simulink model "EV_Modeling"  (R2024b)
(part 7 of 9)

  " Normalization"/3(Current_n) -> Mux2/3
  " Normalization"/1(Temperature_n) -> Mux2/1
  Mux2/1 -> LSTM/1(sequenceinput)
  Divide12/1 -> Add4/1  "Motor_Current"
  Gain5/1 -> Battery_SOC[%]/1, SOC switch/1  "LSTM_LV"
  SOC-Vol/1 -> Voltage_cell/1, " Normalization"/2(Voltage), Vol-R/1, Divide11/1, Vol_pack/1  "Vsoc"
  Zero-Order Hold/1 -> Extended Kalman Filter/1
  Add4/1 -> Gain17/1
  SOC-Temp/1 -> Temperature_cell/1, " Normalization"/1(Temperature)
  SOC switch/1 -> SOC_t-1/1
  Coulomb Counting/1(SOC_CC) -> SOC switch/3, Zero-Order Hold/1
  Zero-Order Hold1/1 -> Extended Kalman Filter/2
  Divide11/1 -> Add4/2  "electric_consumption_Current"
  Extended Kalman Filter/1 -> Gain5/1
  Sum/1 -> [IVD]
  Divide28/1 -> Divide29/1
  From Workspace20/1 -> Divide34/2
  Add1/1 -> Divide33/1
  Constant13/1 -> Divide26/1
  [T_motor] -> Divide38/1
  Divide29/1 -> [T_motor]
  Signal Specification9/1 -> [Motor_radpsec]
  [IVD] -> Saturation1/1
  Gain20/1 -> [Motor_RPM]
  Delay One Step1/1 -> Divide26/2
  Add13/1 -> Divide25/1
  Divide39/1 -> [Electric_Power]
  Add14/1 -> [F_accel]
  [Speed_ms] -> Divide22/2
  [F_resistance] -> Add11/2
  Divide1/1 -> Add1/2  "Motor_Torque[N.m]"
  Divide26/1 -> Add15/4  "F_accel"
  From Workspace14/1 -> Divide29/2
  Divide23/1 -> Add15/3  "F_aero"
  Brake[%]1/1 -> Divide25/2, Divide2/1
  Unit Conversion4/1 -> Signal Specification9/1
  From Workspace21/1 -> Divide35/3
  Divide35/1 -> Divide36/2
  [Motor_RPM] -> 2-D Lookup Table1/1
  Gain23/1 -> Divide39/2
  Compare To Constant3/1 -> Switch1/2
  Divide37/1 -> Gain20/1
  Divide34/1 -> Add14/2
  BPP[%]*MAX_Brake_Force[N]1/1 -> Add14/1  "Brake_Force"
  Constant12/1 -> Divide23/3
  From Workspace22/1 -> Divide37/2
  Constant9/1 -> Divide35/1
  [Motor_efficiency] -> Gain23/1
  Constant10/1 -> Divide35/2
  [Speed_ms] -> Square1/1
  Add11/1 -> Divide28/1
  Square1/1 -> Divide23/2
  2-D Lookup Table1/1 -> [Motor_efficiency]
  Gain14/1 -> BPP[%]*MAX_Brake_Force[N]1/1
  From Workspace19/1 -> Add13/2
  Add15/1 -> [F_resistance]
  Friction_Loss1/1 -> Divide22/1
  [Motor_RPM] -> Signal Specification8/1
  Drag coefficient1/1(C_drag) -> Divide23/1
  [Motor_radpsec] -> Divide38/2
  [Accel_ms2] -> Delay One Step1/1
  From Workspace1/1 -> Divide2/2
  Accel[%]1/1 -> Accel1/1
  Constant8/1 -> Add13/1
  Divide36/1 -> Divide37/1
  [Motor_Power] -> Divide39/1
  MAX Torque1/1 -> Divide27/2, Divide1/1
  Accel1/1 -> Divide1/2
  Divide33/1 -> Divide34/1
  [F_accel] -> Add11/1
  [T_motor] -> 2-D Lookup Table1/2
  Rolling_Loss1/1 -> Switch1/1
  Divide27/1 -> Add1/1  "Motor_Torque[N.m]"
  Saturation1/1 -> Drag coefficient1/1(IVD)
  Switch1/1 -> Add15/1  "F_rolling"
  From Workspace15/1 -> Divide28/2
  Gain13/1 -> Divide27/1
  Constant3/1 -> Switch1/3
  Divide25/1 -> Gain14/1
  Divide22/1 -> Add15/2  "F_friction"
  Divide2/1 -> Gain13/1
  Divide38/1 -> [Motor_Power]
  [Motor_RPM] -> MAX Torque1/1
  Signal Specification8/1 -> Unit Conversion4/1
  From Workspace18/1 -> Divide33/2
  [Speed_ms] -> Divide36/1
  [F_accel] -> Divide15/1
  [Speed_ms] -> Compare To Constant3/1
  Step/1 -> SOC switch/2
